simulink model "week1_4"  (R2020b)
settings: Solver=VariableStepAuto  StartTime=0.0  StopTime=10.0  RelTol=1e-3
settings Model: Creator=Lenovo  LastModifiedBy=Lenovo

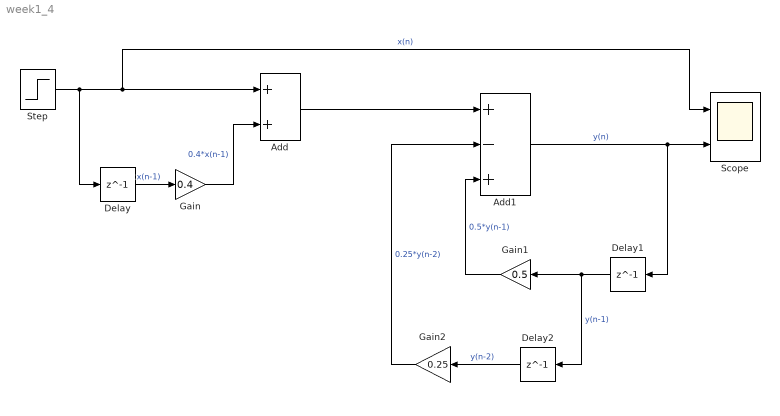
== system week1_4 ==
  Add : Sum
  Add1 : Sum  Inputs=+-+
  Delay : Delay  DelayLength=1  InitialCondition=0
  Delay1 : Delay  DelayLength=1  InitialCondition=0
  Delay2 : Delay  DelayLength=1  InitialCondition=0
  Gain : Gain  Gain=0.4
  Gain1 : Gain  Gain=0.5
  Gain2 : Gain  Gain=0.25
  Scope : Scope  NumInputPorts=2
  Step : Step  SampleTime=0
  wires:
  Step/1 -> Delay/1, Scope/1, Add/1  "x(n)"
  Delay/1 -> Gain/1  "x(n-1)"
  Gain/1 -> Add/2  "0.4*x(n-1)"
  Add/1 -> Add1/1
  Add1/1 -> Delay1/1, Scope/2  "y(n)"
  Delay1/1 -> Delay2/1, Gain1/1  "y(n-1)"
  Gain1/1 -> Add1/3  "0.5*y(n-1)"
  Delay2/1 -> Gain2/1  "y(n-2)"
  Gain2/1 -> Add1/2  "0.25*y(n-2)"
